simulink model "power_controlcurr"  (Simulink 6.0)
settings: Solver=VariableStepDiscrete  SolverMode=SingleTasking  StartTime=0.0  StopTime=100  MaxStep=1e-03  RelTol=1e-3  AbsTol=1e-6
libraries: powerlib x5
settings Model: Creator=patrice  LastModifiedBy=batserve  ExtModeTrigMode=oneshot  ExtModeArmWhenConnect=off  ExtModeAutoUpdateStatusClock=off
settings DataIOCC: LimitDataPoints=off  SignalLoggingName=sigsOut
settings OptimizationCC: BooleanDataType=off
settings DebuggingCC: SolverPrmCheckMsg=none
settings HardwareCC: TargetUnknown=on
settings RTWCC: TemplateMakefile=grt_unix.tmf

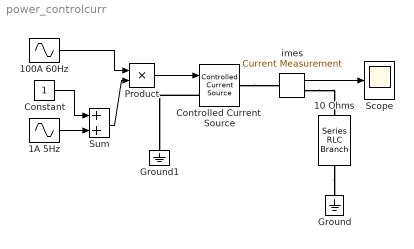
== system power_controlcurr ==
  "10 Ohms " : powerlib/Elements/Series RLC Branch  Orientation=down  PhysicalDomain=powersysdomain  SubClassName=unknown  PortType=p1  LConnTagsString=__new0  RConnTagsString=__new0  Resistance=10  Inductance=0  Capacitance=inf  Measurements=None
  100A 60Hz : Sin  Amplitude=100  Frequency=2*pi*60  SampleTime=0
  1A 5Hz : Sin  Frequency=2*pi*5  SampleTime=0
  Constant : Constant
  Controlled Current  Source : powerlib/Electrical Sources/Controlled Current Source  Description=source block  Initialize=on  Amplitude=0  Phase=0  Frequency=0  Measurements=None
      settings: AttributesFormatString=\n
  Ground : powerlib/Elements/Ground  Orientation=down  PhysicalDomain=powersysdomain  SubClassName=unknown  PortType=p1  LConnTagsString=a
  Ground1 : powerlib/Elements/Ground  Orientation=down  PhysicalDomain=powersysdomain  SubClassName=unknown  PortType=p1  LConnTagsString=a
  Product : Product  SaturateOnIntegerOverflow=on  InputSameDT=on
  Scope : Scope
      settings: TickLabels=on  TimeRange=0.5  YMin=-200  YMax=200  DataFormat=Array
  Sum : Sum  SaturateOnIntegerOverflow=on  InputSameDT=on
  imes : powerlib/Measurements/Current Measurement  Tag=PoWeRsYsTeMmEaSuReMeNt  PhasorSimulation=off  OutputType=Magnitude  PSBequivalent=0
  wires:
  1A 5Hz/1 -> Sum/2
  Constant/1 -> Sum/1
  Sum/1 -> Product/2
  100A 60Hz/1 -> Product/1
  imes/1 -> Scope/1
  Product/1 -> Controlled Current  Source/1
  connections:
  "10 Ohms "/RConn1 -- Ground/LConn1
  imes/RConn1 -- "10 Ohms "/LConn1
  Controlled Current  Source/LConn1 -- Ground1/LConn1
  Controlled Current  Source/RConn1 -- imes/LConn1
